simulink model "nid_cvst_what_is_nid"  (Simulink 10.0)
settings: Solver=FixedStepDiscrete  StartTime=0.0  StopTime=inf  RelTol=1e-3  EnableMultiTasking=on
libraries: vipsnks x4, nid_lib x4
settings Model: Creator=tchikama  LastModifiedBy=bhisma
settings DataIOCC: LimitDataPoints=on  SignalLoggingSaveFormat=ModelDataLogs  SaveOutput=off
settings OptimizationCC: ExpressionDepthLimit=2147483647  SimCompilerOptimization=on
settings DebuggingCC: SolverPrmCheckMsg=warning  FcnCallInpInsideContextMsg=warning  StateNameClashWarn=warning
settings HardwareCC: ProdIntDivRoundTo=Zero  ProdEndianess=LittleEndian  ProdHWDeviceType=Generic->32-bit x86 compatible
settings RTWCC: RTWCompilerOptimization=on
settings CodeAppCC: MaxIdLength=95
settings GRTTargetCC: GeneratePreprocessorConditionals=Disable all
settings ConfigComp: CovExternalEMLEnable=off

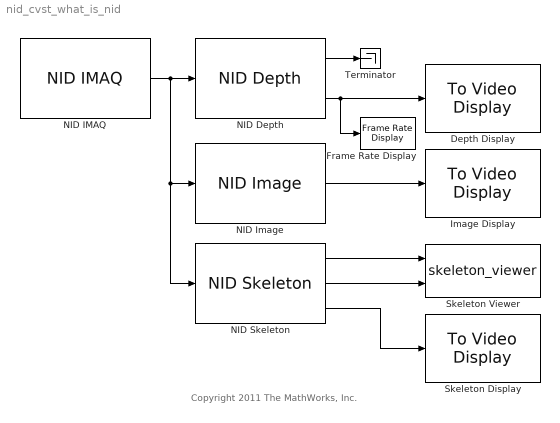
== system nid_cvst_what_is_nid ==
  note: Copyright 2011 The MathWorks, Inc.
  Depth Display : vipsnks/To Video Display  inputType=Obsolete  imagePorts=One multidimensional signal  OutputDevice=On-screen video monitor  fullScreen=off  videoWindowX=1124  videoWindowY=369  saveWindowSize=on  videoWindowWidth=377  videoWindowHeight=292  dataOrg=Column-major  openAtMdlStart=on  isWindowOpen=on
      settings: SourceProductName=Computer Vision Toolbox  SourceProductBaseCode=VP
  Frame Rate Display : vipsnks/Frame Rate Display  UpdateRate=10
      settings: SourceProductName=Computer Vision Toolbox  SourceProductBaseCode=VP
  Image Display : vipsnks/To Video Display  inputType=Obsolete  imagePorts=One multidimensional signal  OutputDevice=On-screen video monitor  fullScreen=off  videoWindowX=1124  videoWindowY=24  saveWindowSize=on  videoWindowWidth=377  videoWindowHeight=292  dataOrg=Column-major  openAtMdlStart=on  isWindowOpen=on
      settings: SourceProductName=Computer Vision Toolbox  SourceProductBaseCode=VP
  NID Depth : nid_lib/NID Depth  depthOutput=Depth  conv_XYZ_RW=off  viewer=on
  NID IMAQ : nid_lib/NID IMAQ  imaq_depth=on  imaq_motion=off  imaq_image=on  view_point=on  imaq_skeleton=on  imaq_ir=off  mirror_image=off  imaq_sample_time=1/30  res_fps=VGA (640x480): 30 FPS  needPsiPose=off  angle=0  angle_read=off  near_mode=off
  NID Image : nid_lib/NID Image  imageOutput=RGB
  NID Skeleton : nid_lib/NID Skeleton  num_of_skeleton_tracking=1  conv_XYZ_RW=on  viewer=on
  Skeleton Display : vipsnks/To Video Display  inputType=Obsolete  imagePorts=One multidimensional signal  OutputDevice=On-screen video monitor  fullScreen=off  videoWindowX=172  videoWindowY=25  saveWindowSize=on  videoWindowWidth=377  videoWindowHeight=292  dataOrg=Column-major  openAtMdlStart=on  isWindowOpen=on
      settings: SourceProductName=Computer Vision Toolbox  SourceProductBaseCode=VP
  Skeleton Viewer : M-S-Function  FunctionName=skeleton_viewer
      mask Display:
      | disp('Skeleton\nViewer')
      | 
      | port_label('input', 1, 'Tracking')
      | port_label('input', 2, 'Skeleton')
  Terminator : Terminator
  wires:
  NID IMAQ/1 -> NID Depth/1, NID Skeleton/1, NID Image/1
  NID Skeleton/1 -> Skeleton Viewer/1
  NID Skeleton/2 -> Skeleton Viewer/2
  NID Skeleton/3 -> Skeleton Display/1
  NID Depth/2 -> Depth Display/1, Frame Rate Display/1
  NID Depth/1 -> Terminator/1
  NID Image/1 -> Image Display/1
